simulink model "DI_cbf_cvxpy"  (R2024a)
settings: Solver=VariableStepAuto  StartTime=0.0  StopTime=Tf  RelTol=1e-3
undefined symbols (not defined in the file): gamma, M, x1_0, x2_0
settings Model: Creator=bumyong  LastModifiedBy=bumyong

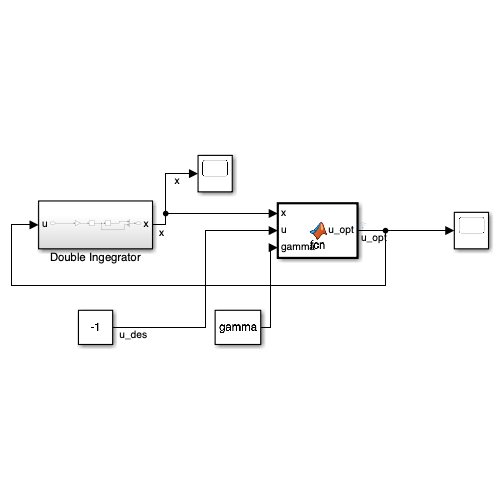
[thumbnail: Simulink's stored preview of the top-level diagram]
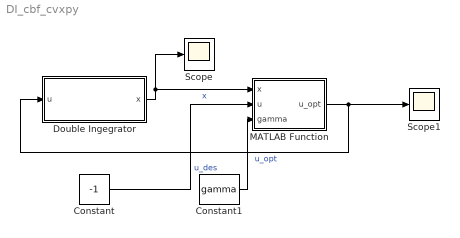
== system DI_cbf_cvxpy ==
  Constant : Constant  Value=-1
  Constant1 : Constant  Value=gamma
  Double Ingegrator : Subsystem
  MATLAB Function : MATLAB Function  TreatAsAtomicUnit=on
  Scope : Scope
  Scope1 : Scope
  wires:
  Double Ingegrator/1(x) -> MATLAB Function/1(x), Scope/1  "x"
  Constant/1 -> MATLAB Function/2(u)  "u_des"
  MATLAB Function/1(u_opt) -> Scope1/1, Double Ingegrator/1(u)  "u_opt"
  Constant1/1 -> MATLAB Function/3(gamma)

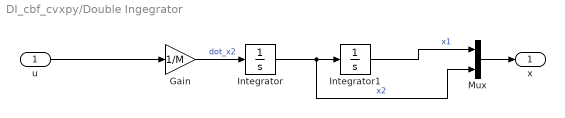
== system DI_cbf_cvxpy/Double Ingegrator ==
  u : Inport
  Gain : Gain  Gain=1/M
  Integrator : Integrator  InitialCondition=x2_0
  Integrator1 : Integrator  InitialCondition=x1_0
  Mux : Mux  Inputs=2
  x : Outport
  wires:
  Gain/1 -> Integrator/1  "dot_x2"
  Integrator/1 -> Mux/2, Integrator1/1  "x2"
  u/1 -> Gain/1
  Integrator1/1 -> Mux/1  "x1"
  Mux/1 -> x/1

== matlab function DI_cbf_cvxpy/MATLAB Function ==
  data: x input; u input; u_opt output; gamma input
function u_opt = fcn(x, u, gamma)
    
    x1 = x(1);
    x2 = x(2);
    u_des = u;

    u_opt = double(0);
 
    coder.extrinsic('py.DI_cbf_cvxpy.DI_cbf_solve')
    

    result = py.DI_cbf_cvxpy.DI_cbf_solve(x1, x2, u_des, gamma);


    u_opt = double(result);
  

end
